simulink model "SysModelPD"  (R2018a)
settings: Solver=VariableStepAuto  StartTime=0.0  StopTime=15.0  RelTol=1e-3
values from neighbouring files (symbols this model uses):
  A = [0      1              0           0 ... (first row only)    [PendulumSSModel.m]    (also in PendulumSSModel_LQR.m = [0                 1                 0                 0; PendulumSSModel_Metric.m = [0                 1                 0                 0; PendulumSSModel_Metric_fxn.m = [0                 1                 0                 0)
  B = [     0 ... (first row only)    [PendulumSSModel.m]    (also in PendulumSSModel_LQR.m = [        0; PendulumSSModel_Metric.m; PendulumSSModel_Metric_fxn.m)
libraries: simulink x1
settings Model: Creator=jcl54  LastModifiedBy=bmo6

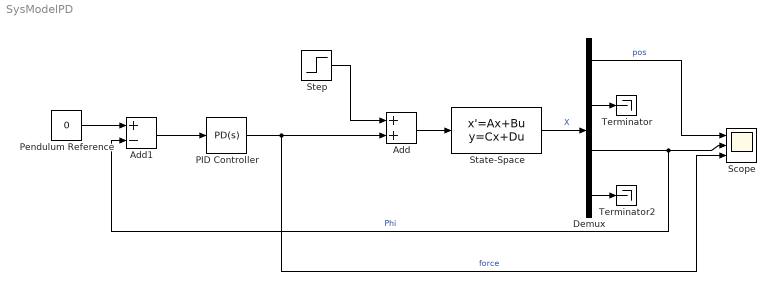
== system SysModelPD ==
  Add : Sum
  Add1 : Sum  Inputs=+-
  Demux : Demux
  PID Controller : simulink/Continuous/PID Controller  Controller=PD  TimeDomain=Continuous-time  SampleTime=-1  IntegratorMethod=Forward Euler  FilterMethod=Forward Euler  Form=Parallel  UseFilter=on  ControllerParametersSource=internal  P=1259.90155075336  I=436.60876367864  D=123.100485397372  N=60968.0156955649  InitialConditionSource=internal  InitialConditionForIntegrator=0  InitialConditionForFilter=0  ExternalReset=none  LimitOutput=on  UpperSaturationLimit=3.9  LowerSaturationLimit=-3.9  LinearizeAsGain=on  AntiWindupMode=none  Kb=1  TrackingMode=off  Kt=1  PParamMin=[]  PParamMax=[]  IParamMin=[]  IParamMax=[]  DParamMin=[]  DParamMax=[]  NParamMin=[]  NParamMax=[]  KbParamMin=[]  KbParamMax=[]  KtParamMin=[]  KtParamMax=[]  POutMin=[]  POutMax=[]  IOutMin=[]  IOutMax=[]  DOutMin=[]  DOutMax=[]  NOutMin=[]  NOutMax=[]  KbOutMin=[]  KbOutMax=[]  KtOutMin=[]  KtOutMax=[]  IntegratorOutMin=[]  IntegratorOutMax=[]  FilterOutMin=[]  FilterOutMax=[]  SumOutMin=[]  SumOutMax=[]  SumI1OutMin=[]  SumI1OutMax=[]  SumI2OutMin=[]  SumI2OutMax=[]  SumI3OutMin=[]  SumI3OutMax=[]  SumDOutMin=[]  SumDOutMax=[]  SaturationOutMin=[]  SaturationOutMax=[]  IntegratorContinuousStateAttributes=''  IntegratorStateMustResolveToSignalObject=off  IntegratorRTWStateStorageClass=Auto  FilterContinuousStateAttributes=''  FilterStateMustResolveToSignalObject=off  FilterRTWStateStorageClass=Auto  DifferentiatorICPrevScaledInput=0  DifferentiatorOutMin=[]  DifferentiatorOutMax=[]  InitialConditionSetting=State (most efficient)  FilterDiffOutCoefMin=[]  FilterDiffOutCoefMax=[]  SumDenOutMin=[]  SumDenOutMax=[]  SumNumOutMin=[]  SumNumOutMax=[]  ReciprocalOutMin=[]  ReciprocalOutMax=[]  DivideOutMin=[]  DivideOutMax=[]  TunerSelectOption=Transfer Function Based (PID Tuner App)
  Pendulum Reference : Constant  Value=0
  Scope : Scope  NumInputPorts=3
  State-Space : StateSpace  A=A  B=B  C=eye(4)  D=zeros(4,1)  InitialCondition=[0,0,0.05,0]  ContinuousStateAttributes={'x','x_dot','phi','phi_dot'}
  Step : Step  Time=3  After=0  SampleTime=0
  Terminator : Terminator
  Terminator2 : Terminator
  wires:
  Step/1 -> Add/1
  Pendulum Reference/1 -> Add1/1
  Add1/1 -> PID Controller/1
  Add/1 -> State-Space/1
  State-Space/1 -> Demux/1  "X"
  Demux/2 -> Terminator/1
  Demux/3 -> Scope/2, Add1/2  "Phi"
  Demux/4 -> Terminator2/1
  Demux/1 -> Scope/1  "pos"
  PID Controller/1 -> Scope/3, Add/2  "force"
